simulink model "disturbance_in_first_second_order_open_close_loop_simulink"  (R2022b)
settings: Solver=VariableStepAuto  StartTime=0.0  StopTime=20  RelTol=1e-3
settings Model: Creator=yasso  LastModifiedBy=yasso

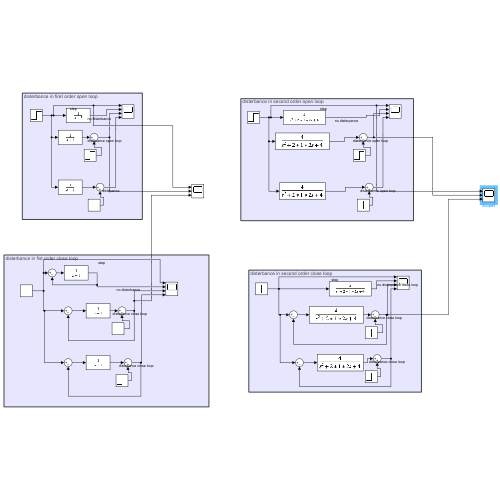
[thumbnail: Simulink's stored preview of the top-level diagram]
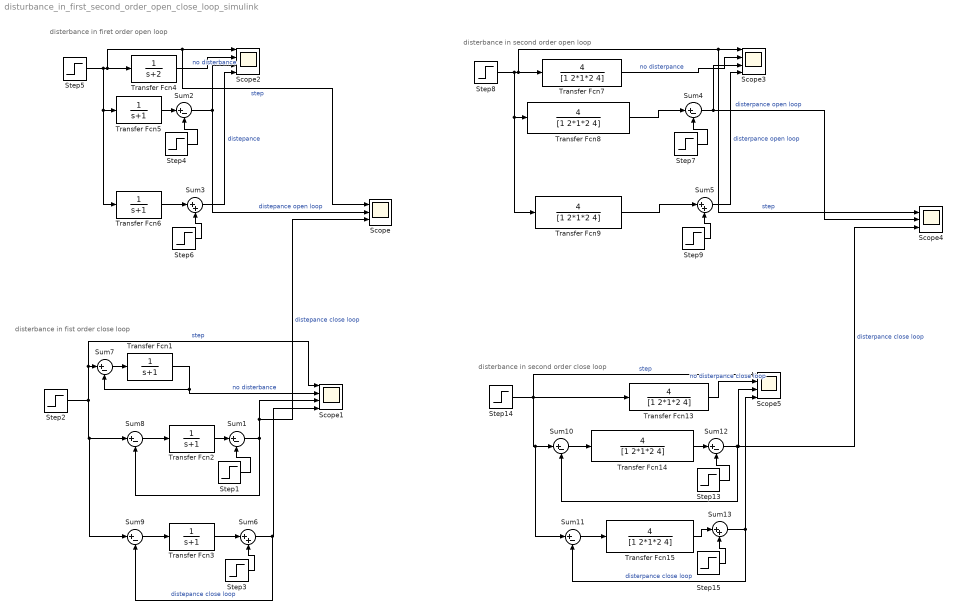
== system disturbance_in_first_second_order_open_close_loop_simulink ==
  note: disterbance in fist order close loop
  note: disterbance in second order open loop
  note: disterbance in firet order open loop
  note: disterbance in second order close loop
  Scope : Scope  NumInputPorts=3
  Scope{1..3,5} (4 alike) : Scope  NumInputPorts=4
  Scope4 : Scope  NumInputPorts=3
  Step{1,3..4,6} (4 alike) : Step  Time=5  After=0.7  SampleTime=0
  Step{7,9,13,15} (4 alike) : Step  Time=10  After=0.7  SampleTime=0
  Step{2,5,8,14} (4 alike) : Step  SampleTime=0
  Sum{1..2,4,7..12} (9 alike) : Sum  Inputs=|+-
  Sum{3,5..6,13} (4 alike) : Sum  Inputs=|++
  Transfer Fcn{1..3,5..6} (5 alike) : TransferFcn  Numerator=1  Denominator=[1 1]
  Transfer Fcn{7..9,13..15} (6 alike) : TransferFcn  Numerator=4  Denominator=[1 2*1*2 4]
  Transfer Fcn4 : TransferFcn  Numerator=1  Denominator=[1 2]
  wires:
  Step5/1 -> Transfer Fcn4/1, Scope/1, Scope2/1, Transfer Fcn6/1, Transfer Fcn5/1  "step"
  Transfer Fcn4/1 -> Scope2/2  "no disterbance"
  Sum2/1 -> Scope2/3, Scope/2  "distepance open loop"
  Step4/1 -> Sum2/2
  Transfer Fcn5/1 -> Sum2/1
  Step6/1 -> Sum3/2
  Transfer Fcn6/1 -> Sum3/1
  Sum3/1 -> Scope2/4  "distepance"
  Sum5/1 -> Scope3/4  "disterpance open loop"
  Transfer Fcn9/1 -> Sum5/1
  Step9/1 -> Sum5/2
  Transfer Fcn8/1 -> Sum4/1
  Step7/1 -> Sum4/2
  Sum4/1 -> Scope3/3, Scope4/2  "disterpance open loop"
  Transfer Fcn7/1 -> Scope3/2  "no disterpance"
  Step8/1 -> Transfer Fcn8/1, Transfer Fcn9/1, Scope4/1, Scope3/1, Transfer Fcn7/1  "step"
  Sum6/1 -> Sum9/2, Scope1/4  "distepance close loop"
  Transfer Fcn3/1 -> Sum6/1
  Transfer Fcn1/1 -> Sum7/2, Scope1/2  "no disterbance"
  Step3/1 -> Sum6/2
  Step1/1 -> Sum1/2
  Step2/1 -> Sum7/1, Scope1/1, Sum9/1, Sum8/1  "step"
  Sum1/1 -> Sum8/2, Scope/3, Scope1/3  "distepance close loop"
  Transfer Fcn2/1 -> Sum1/1
  Sum7/1 -> Transfer Fcn1/1
  Sum8/1 -> Transfer Fcn2/1
  Sum9/1 -> Transfer Fcn3/1
  Sum13/1 -> Sum11/2, Scope5/4  "disterpance close loop"
  Transfer Fcn15/1 -> Sum13/1
  Step15/1 -> Sum13/2
  Transfer Fcn14/1 -> Sum12/1
  Step13/1 -> Sum12/2
  Sum12/1 -> Scope4/3, Scope5/3, Sum10/2  "disterpance close loop"
  Transfer Fcn13/1 -> Scope5/2  "no disterpance close loop"
  Step14/1 -> Sum11/1, Sum10/1, Scope5/1, Transfer Fcn13/1  "step"
  Sum10/1 -> Transfer Fcn14/1
  Sum11/1 -> Transfer Fcn15/1
